simulink model "springmassdamper_sim"  (R2023b)
settings: Solver=VariableStepAuto  StartTime=0.0  StopTime=50  RelTol=1e-3
undefined symbols (not defined in the file): A, den, gain, num
settings Model: Creator=Omistaja  LastModifiedBy=Omistaja

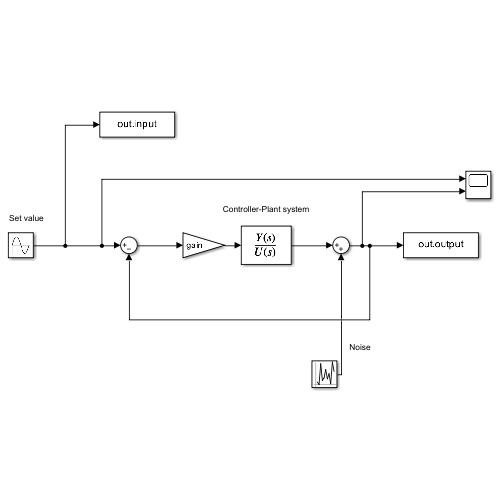
[thumbnail: Simulink's stored preview of the top-level diagram]
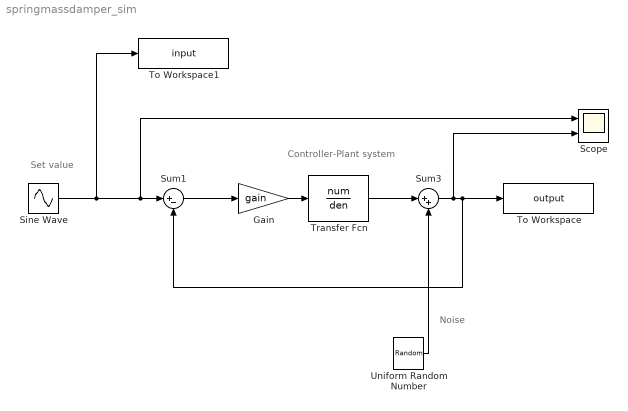
== system springmassdamper_sim ==
  note: Controller-Plant system
  note: Set value
  note: Noise
  Gain : Gain  Gain=gain
  Scope : Scope  NumInputPorts=2
  Sine Wave : Sin  Amplitude=A  SampleTime=0
  Sum1 : Sum  Inputs=|+-
  Sum3 : Sum  Inputs=|++
  To Workspace : ToWorkspace  VariableName=output  SaveFormat=Timeseries  SampleTime=-1
  To Workspace1 : ToWorkspace  VariableName=input  SaveFormat=Timeseries  SampleTime=-1
  Transfer Fcn : TransferFcn  Numerator=num  Denominator=den
  Uniform Random Number : UniformRandomNumber  Minimum=-5  Maximum=5  Seed=5  SampleTime=0.1
  wires:
  Sine Wave/1 -> Sum1/1, Scope/1, To Workspace1/1
  Gain/1 -> Transfer Fcn/1
  Sum1/1 -> Gain/1
  Transfer Fcn/1 -> Sum3/1
  Uniform Random Number/1 -> Sum3/2
  Sum3/1 -> To Workspace/1, Sum1/2, Scope/2
